simulink model "ps3Sim2017"  (R2017b)
settings: Solver=FixedStepAuto  StartTime=0.0  StopTime=inf  FixedStep=0.1  RelTol=1e-3
libraries: vrlib x1
settings Model: SimulationMode=accelerator  Creator=Huib  LastModifiedBy=Huib

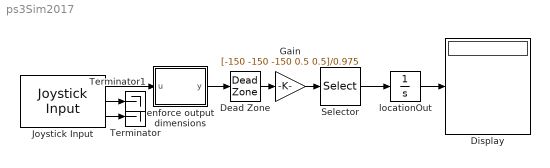
== system ps3Sim2017 ==
  Dead Zone : DeadZone  LowerValue=-0.025  UpperValue=0.025  SaturateOnIntegerOverflow=on
  Display : Display
  Gain : Gain  Gain=[-150 -150 -150 0.5 0.5]/0.975
  Joystick Input : vrlib/Joystick Input  joyid=1  adjustports=on  forcefeed=off
      settings: SourceProductBaseCode=VR
  Selector : Selector  InputPortWidth=5  IndexOptions=Index vector (dialog)  Indices=[2 1 3 4 5]  OutputSizes=1
  Terminator : Terminator
  Terminator1 : Terminator
  enforce output dimensions : MATLAB Function  TreatAsAtomicUnit=on
  locationOut : Integrator  InitialCondition=[1085; 0; 1565; pi; -pi/2]
  wires:
  Joystick Input/1 -> enforce output dimensions/1(u)
  Dead Zone/1 -> Gain/1
  Joystick Input/3 -> Terminator/1
  Joystick Input/2 -> Terminator1/1
  Gain/1 -> Selector/1
  locationOut/1 -> Display/1
  Selector/1 -> locationOut/1
  enforce output dimensions/1(y) -> Dead Zone/1

== matlab function ps3Sim2017/enforce output dimensions ==
  data: u input; y output
function y = fcn(u)
% explicitly output 5 values from analog controller input
% if there are more, only use the first 5, if there are fewer, append zeros
    y = zeros(5,1);
    nAxes = length(u);
    if nAxes >= 5
        y = u(1:5);
    else
        y(1:nAxes) = u;
    end
end
